simulink model "gm_quantized_bpf"  (R2021b)
settings: Solver=VariableStepAuto  StartTime=0.0  StopTime=10.0  RelTol=1e-3
libraries: dsparch4 x1
settings Model: Creator=caccolillo  LastModifiedBy=caccolillo
settings OptimizationCC: BlockReduction=off  ConditionallyExecuteInputs=off
settings DebuggingCC: InheritedTsInSrcMsg=none

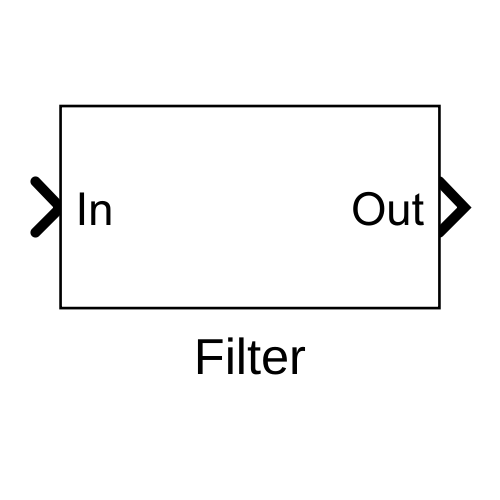
[thumbnail: Simulink's stored preview of the top-level diagram]
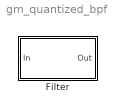
== system gm_quantized_bpf ==
  Filter : Subsystem

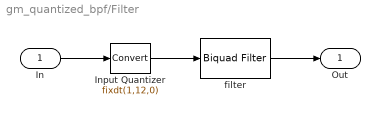
== system gm_quantized_bpf/Filter ==
  In : Inport  OutDataTypeStr=fixdt(1, 12, 0)  PortDimensions=1
  Input Quantizer : DataTypeConversion  OutDataTypeStr=fixdt(1,12,0)  RndMeth=Round  SaturateOnIntegerOverflow=on
  filter : dsparch4/Biquad Filter  FilterSource=Dialog parameters  CoeffSource=Specify via dialog  FilterObject=BQF  IIRFiltStruct=Direct form II  BiQuadCoeffs=[1 0 -1 1 1.65742528830292724 0.815897372432069612;1 0 -1 1 -1.85998922851952742 0.901702779731603621;1 0 -1 1 -1.70469105875488869 0.744422984879922978;1 0 -1 1 1.41335332460150043 0.553995092737038175;1 0 -1 1 -1.61545832429382541 0.654784747265885092;1 0 -1 1 1.28646306613610628 0.420394826751919415]  ScaleValues=[0.885889217627322534;0.885889217627322534;0.799139044168098667;0.799139044168098667;0.759352137722818288;0.759352137722818288;1]  IC=0  ICnum=0  ICden=0  a0Flag=Warning  optimizeScaleValues=on  ScaleValueMode=Specify via input port (g)  InputProcessing=Columns as channels (frame based)  roundingMode=Convergent  overflowMode=on  stageInputMode=Binary point scaling  stageInputWordLength=12  stageInputFracLength=7  stageOutputMode=Binary point scaling  stageOutputWordLength=12  stageOutputFracLength=8  firstCoeffMode=Binary point scaling  firstCoeffWordLength=12  firstCoeffFracLength=10  scaleValueFracLength=11  prodOutputMode=Binary point scaling  prodOutputWordLength=24  prodOutputFracLength=22  denProdOutputFracLength=22  accumMode=Binary point scaling  accumWordLength=40  accumFracLength=22  denAccumFracLength=22  memoryMode=Binary point scaling  memoryWordLength=12  memoryFracLength=12  secondMemoryFracLength=15  outputMode=Binary point scaling  outputWordLength=12  outputFracLength=8
  Out : Outport  SampleTime=0.2
  wires:
  In/1 -> Input Quantizer/1
  Input Quantizer/1 -> filter/1
  filter/1 -> Out/1
